simulink subsystem "PvtSubSys_LATC"  (R2020b)
settings: Solver=VariableStepAuto  StartTime=0.0  StopTime=10.0  RelTol=1e-3
undefined symbols (not defined in the file or in its folder): LCS_PLAN_PreViewIdxNum, LCS_PLAN_PreViewIdxSW_b, P_Global_CharSpd_ms, P_Global_SteeringAngleRatio, P_Global_WheelBase_m, P_LCS_DetNoOverRide_DrvTrq_TH, P_LCS_DetOverRide_DrvTrq_TH, P_LCS_ESS_AngleSlope_Limit, P_LCS_ESS_LogicTest_Enable, P_LCS_ESS_NotActiveFlgDelayTime, P_LCS_ESS_NotActiveFlgDelayTimeSW, P_LCS_ESS_SteerAngleErr, P_LCS_ESS_SteerAngleFilterTime, P_LCS_ESS_TarAngleFilterTime, P_LCS_ESSAngleSW, P_LCS_ESSOverrideTime1, P_LCS_ESSOverrideTime2, P_LCS_ESSOverrideTime3, P_LCS_ESSOverrideValue1, P_LCS_ESSOverrideValue2, P_LCS_IN_Offset_Test_SW, P_LCS_IN_Offset_Test_Value, P_LCS_LATC_AngleFilterTime_s, P_LCS_LATC_CurOffsetCurve_TabX_m, P_LCS_LATC_CurOffsetCurveFliterTime_Tab_s, P_LCS_LATC_CurOffsetVehicleSpdLimitValue_degs, P_LCS_LATC_DeltaEps_Tab_s, P_LCS_LATC_DxOffset_Sw, P_LCS_LATC_ELKAngleSlope_ratio, P_LCS_LATC_ELKMaxLatAcc_ms2, P_LCS_LATC_ESSA0Dis_TabX_m, P_LCS_LATC_ESSAddAngleSlope_Tab_degs, P_LCS_LATC_ESSAESAngleSlope_Tab_degs, P_LCS_LATC_ESSAngleSlope_ratio, P_LCS_LATC_ESSMaxLatAcc_ms2, P_LCS_LATC_LCAngleSlope_ratio, P_LCS_LATC_LCAngleSlope_Tab_degs, P_LCS_LATC_LCCancleMaxLatAcc_ms2, P_LCS_LATC_LCEcoAngleSlope_ratio, P_LCS_LATC_LCEcoAngleSlope_Tab_degs, P_LCS_LATC_LCEcoMaxLatAcc_ms2, P_LCS_LATC_LCKAngleSlope_ratio, P_LCS_LATC_LCKAngleSlope_Tab_degs, P_LCS_LATC_LCKIEAngleSlope_ratio, P_LCS_LATC_LCKIEAngleSlope_Tab_degs, P_LCS_LATC_LCKIEMaxLatAcc_ms2, P_LCS_LATC_LCKMaxLatAcc_ms2, P_LCS_LATC_LCNormalAngleSlope_ratio, P_LCS_LATC_LCNormalAngleSlope_Tab_degs, P_LCS_LATC_LCNormalMaxLatAcc_ms2, P_LCS_LATC_LCSportAngleSlope_ratio, P_LCS_LATC_LCSportAngleSlope_Tab_degs, P_LCS_LATC_LCSportMaxLatAcc_ms2, P_LCS_LATC_LKAAngleSlope_ratio, P_LCS_LATC_LKAAngleSlope_Tab_degs, P_LCS_LATC_LKAMaxLatAcc_ms2, P_LCS_LATC_MatrixQ1_st, P_LCS_LATC_MatrixQ3_st, P_LCS_LATC_MatrixR_st, P_LCS_LATC_MPCDeltaT_s ... (+70)
libraries: simulink x34
(part 2 of 5)

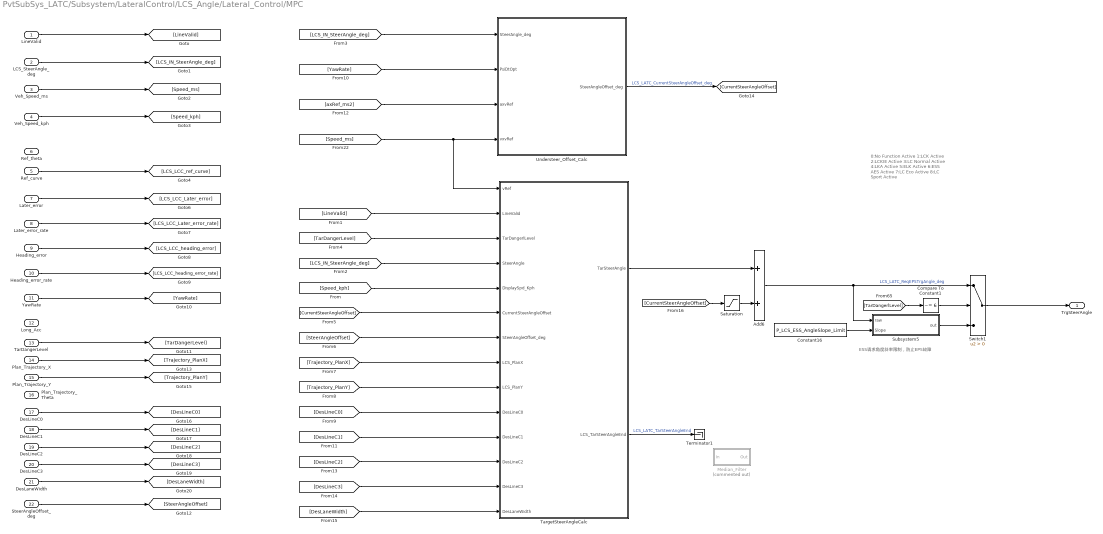
== system PvtSubSys_LATC/Subsystem/LateralControl/LCS_Angle/Lateral_Control/MPC ==
  note: ESS请求角度斜率限制，防止EPS故障
  note: 0:No Function Active
      | 1:LCK Active
      | 2:LCKIE Active
      | 3:LC Normal Active
      | 4:LKA Active
      | 5:ELK Active
      | 6:ESS AES Active
      | 7:LC Eco Active
      | 8:LC Sport Active
  LineValid : Inport
  LCS_SteerAngle_deg : Inport  Port=2
  Veh_Speed_ms : Inport  Port=3
  Veh_Speed_kph : Inport  Port=4
  Ref_curve : Inport  Port=5
  Ref_theta : Inport  Port=6
  Later_error : Inport  Port=7
  Later_error_rate : Inport  Port=8
  Heading_error : Inport  Port=9
  Heading_error_rate : Inport  Port=10
  YawRate : Inport  Port=11
  Long_Acc : Inport  Port=12
  TarDangerLevel : Inport  Port=13
  Plan_Trajectory_X : Inport  Port=14
  Plan_Trajectory_Y : Inport  Port=15
  Plan_Trajectory_Theta : Inport  Port=16
  DesLineC0 : Inport  Port=17
  DesLineC1 : Inport  Port=18
  DesLineC2 : Inport  Port=19
  DesLineC3 : Inport  Port=20
  DesLaneWidth : Inport  Port=21
  SteerAngleOffset_deg : Inport  Port=22
  Add6 : Sum  AccumDataTypeStr=single
  Compare To Constant1 : simulink/Logic and Bit Operations/Compare To Constant  relop=~=  const=6  OutDataTypeStr=boolean
  Constant16 : Constant  Value=P_LCS_ESS_AngleSlope_Limit  OutDataTypeStr=single
  Median_Filter : Subsystem  Commented=on
  Saturation : Saturate  UpperLimit=10  LowerLimit=-10
  Subsystem5 : Subsystem
  Switch1 : Switch  Criteria=u2 > Threshold
  TargetSteerAngleCalc : Subsystem
  Terminator1 : Terminator
  Understeer_Offset_Calc : Subsystem
  TrgSteerAngle : Outport  OutDataTypeStr=single
  wires:
  TarDangerLevel/1 -> [TarDangerLevel]
  YawRate/1 -> [YawRate]
  Later_error_rate/1 -> [LCS_LCC_Later_error_rate]
  Veh_Speed_kph/1 -> [Speed_kph]
  Veh_Speed_ms/1 -> [Speed_ms]
  [axRef_ms2] -> Understeer_Offset_Calc/3(axvRef)
  Understeer_Offset_Calc/1(SteerAngleOffset_deg) -> [CurrentSteerAngleOffset]  "LCS_LATC_CurrentSteerAngleOffset_deg"
  [YawRate] -> Understeer_Offset_Calc/2(PsiDtOpt)
  Heading_error_rate/1 -> [LCS_LCC_heading_error_rate]
  Heading_error/1 -> [LCS_LCC_heading_error]
  Ref_curve/1 -> [LCS_LCC_ref_curve]
  LCS_SteerAngle_deg/1 -> [LCS_IN_SteerAngle_deg]
  [LCS_IN_SteerAngle_deg] -> Understeer_Offset_Calc/1(SteerAngle_deg)
  Later_error/1 -> [LCS_LCC_Later_error]
  LineValid/1 -> [LineValid]
  [Speed_ms] -> TargetSteerAngleCalc/1(vRef), Understeer_Offset_Calc/4(vxvRef)
  [Speed_kph] -> TargetSteerAngleCalc/5(DisplaySpd_Kph)
  [LineValid] -> TargetSteerAngleCalc/2(LineValid)
  [LCS_IN_SteerAngle_deg] -> TargetSteerAngleCalc/4(SteerAngle)
  [TarDangerLevel] -> TargetSteerAngleCalc/3(TarDangerlLevel)
  [CurrentSteerAngleOffset] -> TargetSteerAngleCalc/6(CurrentSteerAngleOffset)
  [SteerAngleOffset] -> TargetSteerAngleCalc/7(SteerAngleOffset_deg)
  SteerAngleOffset_deg/1 -> [SteerAngleOffset]
  [Trajectory_PlanX] -> TargetSteerAngleCalc/8(LCS_PlanX)
  [Trajectory_PlanY] -> TargetSteerAngleCalc/9(LCS_PlanY)
  Plan_Trajectory_X/1 -> [Trajectory_PlanX]
  Plan_Trajectory_Y/1 -> [Trajectory_PlanY]
  [DesLineC0] -> TargetSteerAngleCalc/10(DesLineC0)
  [DesLineC1] -> TargetSteerAngleCalc/11(DesLineC1)
  [DesLineC2] -> TargetSteerAngleCalc/12(DesLineC2)
  [DesLineC3] -> TargetSteerAngleCalc/13(DesLineC3)
  [DesLaneWidth] -> TargetSteerAngleCalc/14(DesLaneWidth)
  DesLineC0/1 -> [DesLineC0]
  DesLineC1/1 -> [DesLineC1]
  DesLineC2/1 -> [DesLineC2]
  DesLineC3/1 -> [DesLineC3]
  DesLaneWidth/1 -> [DesLaneWidth]
  TargetSteerAngleCalc/2(LCS_TarSteerAngleEnd) -> Terminator1/1  "LCS_LATC_TarSteerAngleEnd"
  Subsystem5/1(out) -> Switch1/3
  Constant16/1 -> Subsystem5/2(Slope)
  [CurrentSteerAngleOffset] -> Saturation/1
  Saturation/1 -> Add6/2
  Add6/1 -> Subsystem5/1(raw), Switch1/1  "LCS_LATC_ReqEPSTrgAngle_deg"
  Compare To Constant1/1 -> Switch1/2
  [TarDangerlLevel] -> Compare To Constant1/1
  Switch1/1 -> TrgSteerAngle/1
  TargetSteerAngleCalc/1(TarSteerAngle) -> Add6/1

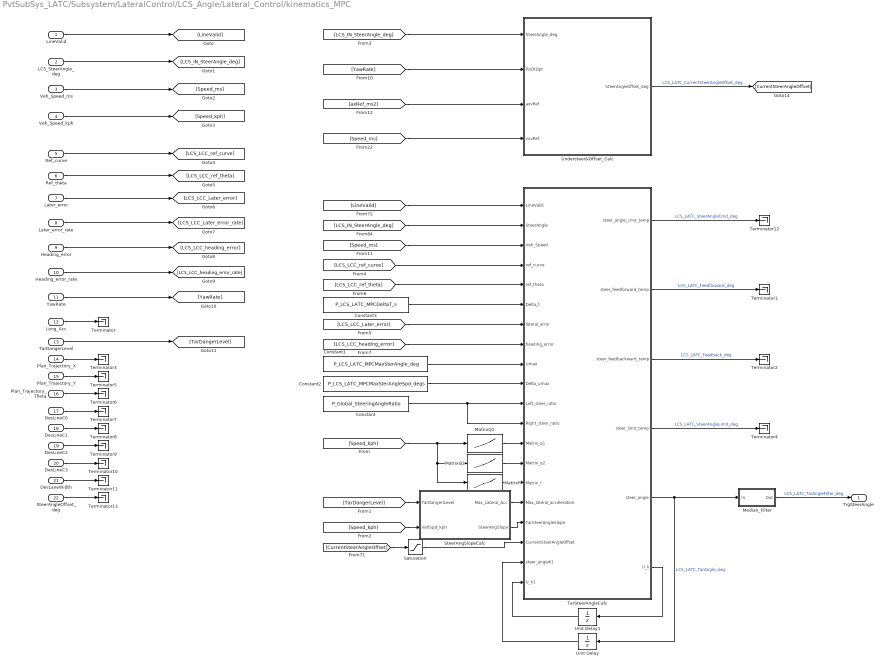
== system PvtSubSys_LATC/Subsystem/LateralControl/LCS_Angle/Lateral_Control/kinematics_MPC ==
  LineValid : Inport
  LCS_SteerAngle_deg : Inport  Port=2
  Veh_Speed_ms : Inport  Port=3
  Veh_Speed_kph : Inport  Port=4
  Ref_curve : Inport  Port=5
  Ref_theta : Inport  Port=6
  Later_error : Inport  Port=7
  Later_error_rate : Inport  Port=8
  Heading_error : Inport  Port=9
  Heading_error_rate : Inport  Port=10
  YawRate : Inport  Port=11
  Long_Acc : Inport  Port=12
  TarDangerLevel : Inport  Port=13
  Plan_Trajectory_X : Inport  Port=14
  Plan_Trajectory_Y : Inport  Port=15
  Plan_Trajectory_Theta : Inport  Port=16
  DesLineC0 : Inport  Port=17
  DesLineC1 : Inport  Port=18
  DesLineC2 : Inport  Port=19
  DesLineC3 : Inport  Port=20
  DesLaneWidth : Inport  Port=21
  SteerAngleOffset_deg : Inport  Port=22
  Constant : Constant  Value=P_Global_SteeringAngleRatio  OutDataTypeStr=single
  Constant1 : Constant  Value=P_LCS_LATC_MPCMaxSterAngle_deg  OutDataTypeStr=single
  Constant2 : Constant  Value=P_LCS_LATC_MPCMaxSterAngleSpd_degs  OutDataTypeStr=single
  Constant3 : Constant  Value=P_LCS_LATC_MPCDeltaT_s  OutDataTypeStr=single
  MatrixQ1 : Lookup_n-D  NumberOfTableDimensions=1  BreakpointsForDimension1=P_LCS_VehicleSpd_TabX_Kph  Table=P_LCS_LATC_MPCMatrixQ1_st  ExtrapMethod=Clip  UseLastTableValue=on  InternalRulePriority=Speed  RndMeth=Simplest  InputSameDT=on
  MatrixQ2 : Lookup_n-D  NumberOfTableDimensions=1  BreakpointsForDimension1=P_LCS_VehicleSpd_TabX_Kph  Table=P_LCS_LATC_MPCMatrixQ2_st  ExtrapMethod=Clip  UseLastTableValue=on  InternalRulePriority=Speed  RndMeth=Simplest  InputSameDT=on
  MatrixR : Lookup_n-D  NumberOfTableDimensions=1  BreakpointsForDimension1=P_LCS_VehicleSpd_TabX_Kph  Table=P_LCS_LATC_MPCMatrixR_st  ExtrapMethod=Clip  UseLastTableValue=on  InternalRulePriority=Speed  RndMeth=Simplest  InputSameDT=on
  Median_Filter : Subsystem
  Saturation : Saturate  UpperLimit=8  LowerLimit=-8  OutDataTypeStr=single
  SteerAngSlopeCalc : Subsystem
  TarSteerAngleCalc : MATLAB Function  TreatAsAtomicUnit=on
  Terminator{,1..13} (14 alike) : Terminator
  Understeer&Offset_Calc : Subsystem
  Unit Delay : UnitDelay  SampleTime=-1  HasFrameUpgradeWarning=on
  Unit Delay1 : UnitDelay  SampleTime=-1  HasFrameUpgradeWarning=on
  TrgSteerAngle : Outport  OutDataTypeStr=single
  wires:
  [LCS_LCC_ref_theta] -> TarSteerAngleCalc/5(ref_theta)
  Ref_theta/1 -> [LCS_LCC_ref_theta]
  Constant3/1 -> TarSteerAngleCalc/6(Delta_t)
  Constant2/1 -> TarSteerAngleCalc/10(Delta_umax)
  Constant1/1 -> TarSteerAngleCalc/9(Umax)
  [LCS_LCC_ref_curve] -> TarSteerAngleCalc/4(ref_curve)
  Unit Delay1/1 -> TarSteerAngleCalc/20(U_k1)
  TarSteerAngleCalc/6(U_k) -> Unit Delay1/1
  Heading_error_rate/1 -> [LCS_LCC_heading_error_rate]
  Long_Acc/1 -> Terminator/1
  Constant/1 -> TarSteerAngleCalc/12(Right_steer_ratio), TarSteerAngleCalc/11(Left_steer_ratio)
  [Speed_kph] -> MatrixQ2/1, MatrixR/1, MatrixQ1/1
  TarSteerAngleCalc/4(steer_limit_temp) -> Terminator4/1  "LCS_LATC_SteerAngleLimit_deg"
  DesLineC3/1 -> Terminator10/1
  MatrixR/1 -> TarSteerAngleCalc/15(Matrix_r)
  [LCS_LCC_Later_error] -> TarSteerAngleCalc/7(lateral_error)
  TarSteerAngleCalc/3(steer_feedbackward_temp) -> Terminator2/1  "LCS_LATC_Feedback_deg"
  [LineValid] -> TarSteerAngleCalc/1(LineValid)
  [Speed_kph] -> SteerAngSlopeCalc/2(VehSpd_kph)
  LCS_SteerAngle_deg/1 -> [LCS_IN_SteerAngle_deg]
  TarSteerAngleCalc/5(steer_angle) -> Median_Filter/1(In), Unit Delay/1  "LCS_LATC_TarAngle_deg"
  [Speed_ms] -> Understeer&Offset_Calc/4(vxvRef)
  Saturation/1 -> TarSteerAngleCalc/18(CurrentSteerAngleOffset)
  [CurrentSteerAngleOffset] -> Saturation/1
  TarDangerLevel/1 -> [TarDangerLevel]
  [LCS_LCC_heading_error] -> TarSteerAngleCalc/8(heading_error)
  [LCS_IN_SteerAngle_deg] -> TarSteerAngleCalc/2(SteerAngle)
  TarSteerAngleCalc/2(steer_feedforward_temp) -> Terminator1/1  "LCS_LATC_Feedforward_deg"
  Median_Filter/1(Out) -> TrgSteerAngle/1  "LCS_LATC_TarAngleFilter_deg"
  [Speed_ms] -> TarSteerAngleCalc/3(Veh_Speed)
  Veh_Speed_ms/1 -> [Speed_ms]
  MatrixQ2/1 -> TarSteerAngleCalc/14(Matrix_q2)
  Later_error/1 -> [LCS_LCC_Later_error]
  Heading_error/1 -> [LCS_LCC_heading_error]
  [YawRate] -> Understeer&Offset_Calc/2(PsiDtOpt)
  LineValid/1 -> [LineValid]
  SteerAngSlopeCalc/2(SteerAngSlope) -> TarSteerAngleCalc/17(TarSteerAngleSlope)
  [LCS_IN_SteerAngle_deg] -> Understeer&Offset_Calc/1(SteerAngle_deg)
  [TarDangerLevel] -> SteerAngSlopeCalc/1(TarDangerlLevel)
  TarSteerAngleCalc/1(steer_angle_cmd_temp) -> Terminator12/1  "LCS_LATC_SteerAngleCmd_deg"
  DesLineC0/1 -> Terminator7/1
  MatrixQ1/1 -> TarSteerAngleCalc/13(Matrix_q1)
  YawRate/1 -> [YawRate]
  [axRef_ms2] -> Understeer&Offset_Calc/3(axvRef)
  Veh_Speed_kph/1 -> [Speed_kph]
  SteerAngSlopeCalc/1(Max_Lateral_Acc) -> TarSteerAngleCalc/16(Max_lateral_acceleration)
  Plan_Trajectory_Theta/1 -> Terminator6/1
  DesLineC2/1 -> Terminator9/1
  DesLineC1/1 -> Terminator8/1
  Later_error_rate/1 -> [LCS_LCC_Later_error_rate]
  Plan_Trajectory_Y/1 -> Terminator5/1
  DesLaneWidth/1 -> Terminator11/1
  Ref_curve/1 -> [LCS_LCC_ref_curve]
  SteerAngleOffset_deg/1 -> Terminator13/1
  Plan_Trajectory_X/1 -> Terminator3/1
  Understeer&Offset_Calc/1(SteerAngleOffset_deg) -> [CurrentSteerAngleOffset]  "LCS_LATC_CurrentSteerAngleOffset_deg"
  Unit Delay/1 -> TarSteerAngleCalc/19(steer_angleK1)

== system PvtSubSys_LATC/Subsystem/LateralControl/LCS_Angle/Motion_Planning/CartesianTrajectory ==
  DesLineValid : Inport
  DesLineC0 : Inport  Port=2
  DesLineC1 : Inport  Port=3
  DesLineC2 : Inport  Port=4
  DesLineC3 : Inport  Port=5
  Veh_Speed_ms : Inport  Port=6
  YawRate : Inport  Port=7
  Veh_Speed_kph : Inport  Port=8
  TarDangerLevel : Inport  Port=9
  Long_Acc : Inport  Port=10
  kapEgo : Inport  Port=11
  Constant : Constant  Value=LCS_PLAN_PreViewIdxSW_b
  Constant1 : Constant  Value=LCS_PLAN_PreViewIdxNum
  DesLineC4 : InportShadow  Port=5
  DesLineC5 : InportShadow  Port=4
  DesLineC6 : InportShadow  Port=2
  FrenetTrajectory : MATLAB Function  TreatAsAtomicUnit=on
  Subsystem1 : Subsystem
  Terminator : Terminator
  Veh_Speed_ms1 : InportShadow  Port=6
  PlanX : Outport
  PlanY : Outport  Port=2
  PlanTheta : Outport  Port=3
  idx : Outport  Port=4
  PreviewX : Outport  Port=5
  PreviewY : Outport  Port=6
  PreviewTheta : Outport  Port=7
  numTraj : Outport  Port=8
  ref_curvature : Outport  Port=9
  ref_theta : Outport  Port=10
  lateral_error : Outport  Port=11
  lateral_error_rate : Outport  Port=12
  heading_error : Outport  Port=13
  heading_error_rate : Outport  Port=14
  wires:
  Constant1/1 -> FrenetTrajectory/13(PreViewIdxNum)
  Constant/1 -> FrenetTrajectory/12(PreViewIdxSW)
  FrenetTrajectory/10(ref_theta) -> ref_theta/1
  DesLineValid/1 -> Terminator/1
  Subsystem1/3(Min_Plan_Dis) -> FrenetTrajectory/9(Min_Plan_Dis)
  kapEgo/1 -> FrenetTrajectory/11(kapEgo)
  DesLineC0/1 -> FrenetTrajectory/1(A0)
  DesLineC1/1 -> FrenetTrajectory/2(A1)
  DesLineC2/1 -> FrenetTrajectory/3(A2)
  DesLineC3/1 -> FrenetTrajectory/4(A3)
  Veh_Speed_ms/1 -> FrenetTrajectory/5(Veh_Speed)
  YawRate/1 -> FrenetTrajectory/6(YawRate)
  FrenetTrajectory/1(PlanX) -> PlanX/1
  FrenetTrajectory/2(PlanY) -> PlanY/1
  FrenetTrajectory/3(PlanTheta) -> PlanTheta/1
  FrenetTrajectory/4(idx) -> idx/1
  FrenetTrajectory/5(PreviewX) -> PreviewX/1
  FrenetTrajectory/6(PreviewY) -> PreviewY/1
  FrenetTrajectory/7(PreviewTheta) -> PreviewTheta/1
  FrenetTrajectory/8(numTraj) -> numTraj/1
  FrenetTrajectory/9(ref_curvature) -> ref_curvature/1
  FrenetTrajectory/11(lateral_error) -> lateral_error/1
  FrenetTrajectory/12(lateral_error_rate) -> lateral_error_rate/1
  FrenetTrajectory/13(heading_error) -> heading_error/1
  FrenetTrajectory/14(heading_error_rate) -> heading_error_rate/1
  Long_Acc/1 -> FrenetTrajectory/10(axEgo)
  Subsystem1/1(Preview_T) -> FrenetTrajectory/7(PreView_T)
  Subsystem1/2(AyDtLimit) -> FrenetTrajectory/8(AyDtLimit)
  TarDangerLevel/1 -> Subsystem1/1(TarDangerLevel)
  Veh_Speed_ms1/1 -> Subsystem1/3(VehSpd_ms)
  Veh_Speed_kph/1 -> Subsystem1/2(Spd_kph)
  DesLineC6/1 -> Subsystem1/4(LCS_IN_desLaneA0)
  DesLineC5/1 -> Subsystem1/5(LCS_IN_desLaneA2)
  DesLineC4/1 -> Subsystem1/6(LCS_IN_desLaneA3)

== system PvtSubSys_LATC/Subsystem/LateralControl/LCS_Angle/Motion_Planning/CartesianTrajectory_MPC ==
  DesLineValid : Inport
  DesLineC0 : Inport  Port=2
  DesLineC1 : Inport  Port=3
  DesLineC2 : Inport  Port=4
  DesLineC3 : Inport  Port=5
  Veh_Speed_ms : Inport  Port=6
  YawRate : Inport  Port=7
  Veh_Speed_kph : Inport  Port=8
  TarDangerLevel : Inport  Port=9
  Long_Acc : Inport  Port=10
  kapEgo : Inport  Port=11
  CartesianTrajectory : MATLAB Function  TreatAsAtomicUnit=on
  Constant10 : Constant  Value=P_LCS_PLAN_DisFac_Tab_ratio  OutDataTypeStr=single
  Constant2 : Constant  Value=P_LCS_PLAN_MinDis_m  OutDataTypeStr=single
  Ground{,1..10} (11 alike) : Ground
  Subsystem : Subsystem
  Terminator{2..7,9..10} (8 alike) : Terminator
  Veh_Speed_ms1 : InportShadow  Port=6
  PlanX : Outport
  PlanY : Outport  Port=2
  PlanTheta : Outport  Port=3
  idx : Outport  Port=4
  PreviewX : Outport  Port=5
  PreviewY : Outport  Port=6
  PreviewTheta : Outport  Port=7
  numTraj : Outport  Port=8
  ref_curvature : Outport  Port=9
  ref_theta : Outport  Port=10
  lateral_error : Outport  Port=11
  lateral_error_rate : Outport  Port=12
  heading_error : Outport  Port=13
  heading_error_rate : Outport  Port=14
  wires:
  Ground10/1 -> ref_theta/1
  CartesianTrajectory/6(planLength) -> Terminator10/1  "LCS_LATC_PlanLength"
  CartesianTrajectory/5(LoopNum) -> numTraj/1
  CartesianTrajectory/7(Ay) -> Terminator4/1
  CartesianTrajectory/11(break_AyDtValue) -> Terminator6/1
  CartesianTrajectory/2(planY) -> PlanY/1
  CartesianTrajectory/1(planX) -> PlanX/1
  CartesianTrajectory/3(planValid) -> Terminator9/1
  CartesianTrajectory/8(AyDt) -> Terminator5/1  "LCS_LATC_PlanAyDt"
  CartesianTrajectory/9(break_Flg) -> Terminator3/1
  CartesianTrajectory/4(planT) -> Terminator7/1  "LCS_LATC_PlanT"
  CartesianTrajectory/10(break_AyValue) -> Terminator2/1
  Ground/1 -> PlanTheta/1
  Ground1/1 -> idx/1
  Ground2/1 -> PreviewX/1
  Ground3/1 -> PreviewY/1
  Ground4/1 -> PreviewTheta/1
  Ground5/1 -> ref_curvature/1
  Ground6/1 -> lateral_error/1
  Ground7/1 -> lateral_error_rate/1
  Ground8/1 -> heading_error/1
  Ground9/1 -> heading_error_rate/1
  Veh_Speed_ms/1 -> CartesianTrajectory/1(vEgo)
  DesLineC0/1 -> Subsystem/4(DesLineC0), CartesianTrajectory/8(TarLineC0)
  DesLineC1/1 -> Subsystem/5(DesLineC1), CartesianTrajectory/7(TarLineC1)
  DesLineC2/1 -> Subsystem/6(DesLineC2), CartesianTrajectory/6(TarLineC2)
  DesLineC3/1 -> Subsystem/7(DesLineC3), CartesianTrajectory/5(TarLineC3)
  kapEgo/1 -> CartesianTrajectory/2(kapEgo)
  Long_Acc/1 -> CartesianTrajectory/3(axEgo)
  DesLineValid/1 -> CartesianTrajectory/4(TarLineValid)
  Subsystem/1(Plan_ayDtLimit) -> CartesianTrajectory/9(ayDtLimit)
  Subsystem/2(Plan_FinalpreDis) -> CartesianTrajectory/10(PreDis)
  Constant10/1 -> CartesianTrajectory/11(Dis_Fac)
  Constant2/1 -> CartesianTrajectory/12(Min_PlanDis)
  TarDangerLevel/1 -> Subsystem/1(TarDangerlLevel)
  Veh_Speed_ms1/1 -> Subsystem/3(Veh_Speed_ms)
  Veh_Speed_kph/1 -> Subsystem/2(vDisplay_Kph)

== system PvtSubSys_LATC/Subsystem/LateralControl/LCS_Angle/Motion_Planning/FrenetTrajectory ==
  DesLineValid : Inport
  DesLineC0 : Inport  Port=2
  DesLineC1 : Inport  Port=3
  DesLineC2 : Inport  Port=4
  DesLineC3 : Inport  Port=5
  Veh_Speed_ms : Inport  Port=6
  YawRate : Inport  Port=7
  Veh_Speed_kph : Inport  Port=8
  TarDangerLevel : Inport  Port=9
  Long_Acc : Inport  Port=10
  kapEgo : Inport  Port=11
  Constant : Constant  Value=LCS_PLAN_PreViewIdxSW_b
  Constant1 : Constant  Value=LCS_PLAN_PreViewIdxNum
  DesLineC4 : InportShadow  Port=2
  DesLineC5 : InportShadow  Port=4
  DesLineC6 : InportShadow  Port=5
  FrenetTrajectory : MATLAB Function  TreatAsAtomicUnit=on
  Subsystem : Subsystem
  Terminator : Terminator
  Terminator1 : Terminator
  Terminator2 : Terminator
  Veh_Speed_ms1 : InportShadow  Port=6
  PlanX : Outport
  PlanY : Outport  Port=2
  PlanTheta : Outport  Port=3
  idx : Outport  Port=4
  PreviewX : Outport  Port=5
  PreviewY : Outport  Port=6
  PreviewTheta : Outport  Port=7
  numTraj : Outport  Port=8
  ref_curvature : Outport  Port=9
  ref_theta : Outport  Port=10
  lateral_error : Outport  Port=11
  lateral_error_rate : Outport  Port=12
  heading_error : Outport  Port=13
  heading_error_rate : Outport  Port=14
  wires:
  Constant1/1 -> FrenetTrajectory/11(PreViewIdxNum)
  Constant/1 -> FrenetTrajectory/10(PreViewIdxSW)
  FrenetTrajectory/10(ref_theta) -> ref_theta/1
  DesLineValid/1 -> Terminator2/1
  Subsystem/3(Min_Plan_Dis) -> FrenetTrajectory/9(Min_Plan_Dis)
  kapEgo/1 -> Terminator1/1
  DesLineC6/1 -> Subsystem/6(LCS_IN_desLaneA3)
  DesLineC5/1 -> Subsystem/5(LCS_IN_desLaneA2)
  DesLineC4/1 -> Subsystem/4(LCS_IN_desLaneA0)
  Veh_Speed_kph/1 -> Subsystem/2(Spd_kph)
  Veh_Speed_ms1/1 -> Subsystem/3(VehSpd_ms)
  TarDangerLevel/1 -> Subsystem/1(TarDangerLevel)
  Subsystem/2(AyDtLimit) -> FrenetTrajectory/8(AyDtLimit)
  Subsystem/1(Preview_T) -> FrenetTrajectory/7(PreView_T)
  Long_Acc/1 -> Terminator/1
  FrenetTrajectory/14(heading_error_rate) -> heading_error_rate/1
  FrenetTrajectory/13(heading_error) -> heading_error/1
  FrenetTrajectory/12(lateral_error_rate) -> lateral_error_rate/1
  FrenetTrajectory/11(lateral_error) -> lateral_error/1
  FrenetTrajectory/9(ref_curvature) -> ref_curvature/1
  FrenetTrajectory/8(numTraj) -> numTraj/1
  FrenetTrajectory/7(PreviewTheta) -> PreviewTheta/1
  FrenetTrajectory/6(PreviewY) -> PreviewY/1
  FrenetTrajectory/5(PreviewX) -> PreviewX/1
  FrenetTrajectory/4(idx) -> idx/1
  FrenetTrajectory/3(PlanTheta) -> PlanTheta/1
  FrenetTrajectory/2(PlanY) -> PlanY/1
  FrenetTrajectory/1(PlanX) -> PlanX/1
  YawRate/1 -> FrenetTrajectory/6(YawRate)
  Veh_Speed_ms/1 -> FrenetTrajectory/5(Veh_Speed)
  DesLineC3/1 -> FrenetTrajectory/4(A3)
  DesLineC2/1 -> FrenetTrajectory/3(A2)
  DesLineC1/1 -> FrenetTrajectory/2(A1)
  DesLineC0/1 -> FrenetTrajectory/1(A0)

== system PvtSubSys_LATC/Subsystem/LateralControl/LCS_Angle/Motion_Planning/FrenetTrajectory_Lateral ==
  DesLineValid : Inport
  DesLineC0 : Inport  Port=2
  DesLineC1 : Inport  Port=3
  DesLineC2 : Inport  Port=4
  DesLineC3 : Inport  Port=5
  Veh_Speed_ms : Inport  Port=6
  YawRate : Inport  Port=7
  Veh_Speed_kph : Inport  Port=8
  TarDangerLevel : Inport  Port=9
  Long_Acc : Inport  Port=10
  kapEgo : Inport  Port=11
  Constant : Constant  Value=LCS_PLAN_PreViewIdxSW_b
  Constant1 : Constant  Value=LCS_PLAN_PreViewIdxNum
  DesLineC4 : InportShadow  Port=2
  DesLineC5 : InportShadow  Port=4
  DesLineC6 : InportShadow  Port=5
  FrenetTrajectory_Lateral : MATLAB Function  TreatAsAtomicUnit=on
  Subsystem1 : Subsystem
  Terminator : Terminator
  Terminator1 : Terminator
  Terminator2 : Terminator
  Veh_Speed_ms1 : InportShadow  Port=6
  PlanX : Outport
  PlanY : Outport  Port=2
  PlanTheta : Outport  Port=3
  idx : Outport  Port=4
  PreviewX : Outport  Port=5
  PreviewY : Outport  Port=6
  PreviewTheta : Outport  Port=7
  numTraj : Outport  Port=8
  ref_curvature : Outport  Port=9
  ref_theta : Outport  Port=10
  lateral_error : Outport  Port=11
  lateral_error_rate : Outport  Port=12
  heading_error : Outport  Port=13
  heading_error_rate : Outport  Port=14
  wires:
  Constant1/1 -> FrenetTrajectory_Lateral/12(PreViewIdxNum)
  Constant/1 -> FrenetTrajectory_Lateral/11(PreViewIdxSW)
  FrenetTrajectory_Lateral/10(ref_theta) -> ref_theta/1
  Subsystem1/3(Min_Plan_Dis) -> FrenetTrajectory_Lateral/10(Min_Plan_Dis)
  DesLineValid/1 -> Terminator2/1
  kapEgo/1 -> Terminator1/1
  DesLineC6/1 -> Subsystem1/6(LCS_IN_desLaneA3)
  DesLineC5/1 -> Subsystem1/5(LCS_IN_desLaneA2)
  DesLineC0/1 -> FrenetTrajectory_Lateral/1(A0)
  DesLineC1/1 -> FrenetTrajectory_Lateral/2(A1)
  DesLineC2/1 -> FrenetTrajectory_Lateral/3(A2)
  DesLineC3/1 -> FrenetTrajectory_Lateral/4(A3)
  Veh_Speed_ms/1 -> FrenetTrajectory_Lateral/5(Veh_Speed)
  YawRate/1 -> FrenetTrajectory_Lateral/6(YawRate)
  FrenetTrajectory_Lateral/1(PlanX) -> PlanX/1
  FrenetTrajectory_Lateral/2(PlanY) -> PlanY/1
  FrenetTrajectory_Lateral/3(PlanTheta) -> PlanTheta/1
  FrenetTrajectory_Lateral/4(idx) -> idx/1
  FrenetTrajectory_Lateral/5(PreviewX) -> PreviewX/1
  FrenetTrajectory_Lateral/6(PreviewY) -> PreviewY/1
  FrenetTrajectory_Lateral/7(PreviewTheta) -> PreviewTheta/1
  FrenetTrajectory_Lateral/8(numTraj) -> numTraj/1
  FrenetTrajectory_Lateral/9(ref_curvature) -> ref_curvature/1
  FrenetTrajectory_Lateral/11(lateral_error) -> lateral_error/1
  FrenetTrajectory_Lateral/12(lateral_error_rate) -> lateral_error_rate/1
  FrenetTrajectory_Lateral/13(heading_error) -> heading_error/1
  FrenetTrajectory_Lateral/14(heading_error_rate) -> heading_error_rate/1
  Long_Acc/1 -> Terminator/1
  Subsystem1/1(Preview_T) -> FrenetTrajectory_Lateral/8(PreView_T)
  Subsystem1/2(AyDtLimit) -> FrenetTrajectory_Lateral/9(AyDtLimit)
  TarDangerLevel/1 -> FrenetTrajectory_Lateral/7(TarDangerlLevel), Subsystem1/1(TarDangerLevel)
  Veh_Speed_ms1/1 -> Subsystem1/3(VehSpd_ms)
  Veh_Speed_kph/1 -> Subsystem1/2(Spd_kph)
  DesLineC4/1 -> Subsystem1/4(LCS_IN_desLaneA0)

== system PvtSubSys_LATC/Subsystem/LateralControl/LCS_Angle/OverRideDetect/LP filter4 ==
  note: deltaT = time(signal) - time(signal[-1]);
      |    alpha = 1/(1/2/pi/deltaT/fc + 1);
      |    result = alpha * signal + (1 - alpha) * LastValue;
  Raw : Inport
  TorqFilterTime : Inport  Port=2
  enable : Inport  Port=3
  Add : Sum
  Add1 : Sum  Inputs=+-
  Data Type Conversion : DataTypeConversion  OutDataTypeStr=single
  Memory2 : Memory  InheritSampleTime=on
  Product2 : Product  Inputs=*/  RndMeth=Zero
  Product3 : Product  RndMeth=Zero
  Product4 : Product  Inputs=*//  RndMeth=Zero
  Product5 : Product  RndMeth=Zero
  Sum1 : Sum  Inputs=++|
  Switch1 : Switch  Criteria=u2 ~= 0
  Weight/N1 : Constant  Value=0.1591549431  OutDataTypeStr=single
  Weight/N2 : Constant  OutDataTypeStr=single
  Weight/N3 : Constant  Value=0.02  OutDataTypeStr=single
  output : Outport
  wires:
  TorqFilterTime/1 -> Product4/3
  Product4/1 -> Add/1
  Weight/N3/1 -> Product4/2
  Memory2/1 -> Data Type Conversion/1
  enable/1 -> Switch1/2
  Raw/1 -> Product3/2, Switch1/3
  Switch1/1 -> output/1, Memory2/1
  Weight/N1/1 -> Product4/1
  Weight/N2/1 -> Add1/1, Product2/1, Add/2
  Add/1 -> Product2/2
  Product2/1 -> Product3/1, Add1/2
  Product3/1 -> Sum1/2
  Add1/1 -> Product5/2
  Product5/1 -> Sum1/1
  Sum1/1 -> Switch1/1
  Data Type Conversion/1 -> Product5/1

== system PvtSubSys_LATC/Subsystem/LateralControl/LCS_Angle/OverRideDetect/Subsystem17 ==
  In1 : Inport
  Add : Sum
  Constant : Constant  Value=Ts
  Constant1 : Constant  Value=0
  Constant2 : Constant  Value=Max
  Max : MinMax  Inputs=2
  Switch : Switch  Criteria=u2 ~= 0
  Unit Delay : UnitDelay  SampleTime=-1  HasFrameUpgradeWarning=on
  Out1 : Outport
  wires:
  Switch/1 -> Max/1
  Constant2/1 -> Max/2
  Max/1 -> Out1/1, Unit Delay/1
  Add/1 -> Switch/1
  Constant1/1 -> Switch/3
  Constant/1 -> Add/2
  In1/1 -> Switch/2
  Unit Delay/1 -> Add/1

== system PvtSubSys_LATC/Subsystem/LateralControl/LCS_Angle/OverRideDetect/Subsystem4 ==
  In1 : Inport
  Add : Sum
  Constant : Constant  Value=Ts
  Constant1 : Constant  Value=0
  Constant2 : Constant  Value=Max
  Max : MinMax  Inputs=2
  Switch : Switch  Criteria=u2 ~= 0
  Unit Delay : UnitDelay  SampleTime=-1  HasFrameUpgradeWarning=on
  Out1 : Outport
  wires:
  Unit Delay/1 -> Add/1
  In1/1 -> Switch/2
  Constant/1 -> Add/2
  Constant1/1 -> Switch/3
  Add/1 -> Switch/1
  Max/1 -> Unit Delay/1, Out1/1
  Constant2/1 -> Max/2
  Switch/1 -> Max/1

== system PvtSubSys_LATC/Subsystem/LateralControl/LCS_Angle/Lateral_Control/Dynamic_Model_LQR/Median_Filter ==
  In : Inport
  Constant11 : Constant  Value=P_LCS_LATC_TarAngleFliterWindowSize - single(2)  OutDataTypeStr=single
  Divide1 : Product  Inputs=*/
  Max of Elements1 : MinMax  Function=max
  MinMax2 : MinMax
  Minus1 : Sum  Inputs=--+
  Sum of Elements1 : Sum  Inputs=+
  Tapped Delay1 : simulink/Discrete/Tapped Delay  vinit=0.0  samptime=-1  NumDelays=P_LCS_LATC_TarAngleFliterWindowSize-1  DelayOrder=Newest  includeCurrent=on
  Out : Outport
  wires:
  Max of Elements1/1 -> Minus1/2
  Divide1/1 -> Out/1
  Minus1/1 -> Divide1/1
  In/1 -> Tapped Delay1/1
  MinMax2/1 -> Minus1/1
  Sum of Elements1/1 -> Minus1/3
  Tapped Delay1/1 -> Max of Elements1/1, MinMax2/1, Sum of Elements1/1
  Constant11/1 -> Divide1/2

== system PvtSubSys_LATC/Subsystem/LateralControl/LCS_Angle/Lateral_Control/Dynamic_Model_LQR/SteerAngSlopeCalc ==
  note: 换道状态切换检测
  note: 0:No Function Active
      | 1:LCK Active
      | 2:LCKIE Active
      | 3:LC Normal Active
      | 4:LKA Active
      | 5:ELK Active
      | 6:ESS AES Active
      | 7:LC Eco Active
      | 8:LC Sport Active
      | 9:LC cancel
  TarDangerlLevel : Inport
  VehSpd_kph : Inport  Port=2
  Constant : Constant  Value=0.4  OutDataTypeStr=single
  Constant1 : Constant  Value=1.5  OutDataTypeStr=single
  Constant2 : Constant  Value=P_LCS_LATC_StateHoldTime_st  OutDataTypeStr=uint16
  Constant3 : Constant  Value=0.02
  Constant4 : Constant  Value=0.4  OutDataTypeStr=single
  Constant5 : Constant  Value=1.5  OutDataTypeStr=single
  Data Type Conversion : DataTypeConversion  OutDataTypeStr=single
  Data Type Conversion1 : DataTypeConversion  OutDataTypeStr=single
  ELK Active : Lookup_n-D  NumberOfTableDimensions=1  BreakpointsForDimension1=P_LCS_VehicleSpd_TabX_Kph  Table=P_LCS_LATC_ELKAngleSlope_ratio  ExtrapMethod=Clip  InternalRulePriority=Speed  RndMeth=Simplest  InputSameDT=on
  ELK_MaxAy : Lookup_n-D  NumberOfTableDimensions=1  BreakpointsForDimension1=P_LCS_VehicleSpd_TabX_Kph  Table=P_LCS_LATC_ELKMaxLatAcc_ms2  ExtrapMethod=Clip  InternalRulePriority=Speed  RndMeth=Simplest  InputSameDT=on
  ESS AES Active : Lookup_n-D  NumberOfTableDimensions=1  BreakpointsForDimension1=P_LCS_VehicleSpd_TabX_Kph  Table=P_LCS_LATC_ESSAngleSlope_ratio  ExtrapMethod=Clip  InternalRulePriority=Speed  RndMeth=Simplest  InputSameDT=on
  ESS AES_MaxAy : Lookup_n-D  NumberOfTableDimensions=1  BreakpointsForDimension1=P_LCS_VehicleSpd_TabX_Kph  Table=P_LCS_LATC_ESSMaxLatAcc_ms2  ExtrapMethod=Clip  InternalRulePriority=Speed  RndMeth=Simplest  InputSameDT=on
  LC Cancel : Lookup_n-D  NumberOfTableDimensions=1  BreakpointsForDimension1=P_LCS_VehicleSpd_TabX_Kph  Table=P_LCS_LATC_LCAngleSlope_ratio  ExtrapMethod=Clip  InternalRulePriority=Speed  RndMeth=Simplest  InputSameDT=on
  LCK/IE TO LC_Eco : Lookup_n-D  NumberOfTableDimensions=1  BreakpointsForDimension1=P_LCS_VehicleSpd_TabX_Kph  Table=P_LCS_LATC_LCEcoAngleSlope_ratio  ExtrapMethod=Clip  InternalRulePriority=Speed  RndMeth=Simplest  InputSameDT=on
  LCK/IE TO LC_Nomal : Lookup_n-D  NumberOfTableDimensions=1  BreakpointsForDimension1=P_LCS_VehicleSpd_TabX_Kph  Table=P_LCS_LATC_LCNormalAngleSlope_ratio  ExtrapMethod=Clip  InternalRulePriority=Speed  RndMeth=Simplest  InputSameDT=on
  LCK/IE TO LC_Sport : Lookup_n-D  NumberOfTableDimensions=1  BreakpointsForDimension1=P_LCS_VehicleSpd_TabX_Kph  Table=P_LCS_LATC_LCSportAngleSlope_ratio  ExtrapMethod=Clip  InternalRulePriority=Speed  RndMeth=Simplest  InputSameDT=on
  LCKIEMaxAy : Lookup_n-D  NumberOfTableDimensions=1  BreakpointsForDimension1=P_LCS_VehicleSpd_TabX_Kph  Table=P_LCS_LATC_LCKIEMaxLatAcc_ms2  ExtrapMethod=Clip  InternalRulePriority=Speed  RndMeth=Simplest  InputSameDT=on
  LCKIE_Active : Lookup_n-D  NumberOfTableDimensions=1  BreakpointsForDimension1=P_LCS_VehicleSpd_TabX_Kph  Table=P_LCS_LATC_LCKIEAngleSlope_ratio  ExtrapMethod=Clip  InternalRulePriority=Speed  RndMeth=Simplest  InputSameDT=on
  LCKMaxAy : Lookup_n-D  NumberOfTableDimensions=1  BreakpointsForDimension1=P_LCS_VehicleSpd_TabX_Kph  Table=P_LCS_LATC_LCKMaxLatAcc_ms2  ExtrapMethod=Clip  InternalRulePriority=Speed  RndMeth=Simplest  InputSameDT=on
  LCNomal_MaxAy : Lookup_n-D  NumberOfTableDimensions=1  BreakpointsForDimension1=P_LCS_VehicleSpd_TabX_Kph  Table=P_LCS_LATC_LCNormalMaxLatAcc_ms2  ExtrapMethod=Clip  InternalRulePriority=Speed  RndMeth=Simplest  InputSameDT=on
  LC_CancelMaxAy : Lookup_n-D  NumberOfTableDimensions=1  BreakpointsForDimension1=P_LCS_VehicleSpd_TabX_Kph  Table=P_LCS_LATC_LCCancleMaxLatAcc_ms2  ExtrapMethod=Clip  InternalRulePriority=Speed  RndMeth=Simplest  InputSameDT=on
  LC_Eco_MaxAy : Lookup_n-D  NumberOfTableDimensions=1  BreakpointsForDimension1=P_LCS_VehicleSpd_TabX_Kph  Table=P_LCS_LATC_LCEcoMaxLatAcc_ms2  ExtrapMethod=Clip  InternalRulePriority=Speed  RndMeth=Simplest  InputSameDT=on
  LC_SportMaxAy : Lookup_n-D  NumberOfTableDimensions=1  BreakpointsForDimension1=P_LCS_VehicleSpd_TabX_Kph  Table=P_LCS_LATC_LCSportMaxLatAcc_ms2  ExtrapMethod=Clip  InternalRulePriority=Speed  RndMeth=Simplest  InputSameDT=on
  LKA Active : Lookup_n-D  NumberOfTableDimensions=1  BreakpointsForDimension1=P_LCS_VehicleSpd_TabX_Kph  Table=P_LCS_LATC_LKAAngleSlope_ratio  ExtrapMethod=Clip  InternalRulePriority=Speed  RndMeth=Simplest  InputSameDT=on
  LKA_MaxAy : Lookup_n-D  NumberOfTableDimensions=1  BreakpointsForDimension1=P_LCS_VehicleSpd_TabX_Kph  Table=P_LCS_LATC_LKAMaxLatAcc_ms2  ExtrapMethod=Clip  InternalRulePriority=Speed  RndMeth=Simplest  InputSameDT=on
  MATLAB Function3 : MATLAB Function  TreatAsAtomicUnit=on
  Merge : Merge
  Min : MinMax  Inputs=2
  Multiport Switch1 : MultiPortSwitch  DataPortOrder=Zero-based contiguous  Inputs=11  zeroidx=on
  Multiport Switch2 : MultiPortSwitch  DataPortOrder=Zero-based contiguous  Inputs=11  zeroidx=on
  No Function 2 LCK : Lookup_n-D  NumberOfTableDimensions=1  BreakpointsForDimension1=P_LCS_VehicleSpd_TabX_Kph  Table=P_LCS_LATC_LCKAngleSlope_ratio  ExtrapMethod=Clip  InternalRulePriority=Speed  RndMeth=Simplest  InputSameDT=on
  Product : Product
  Switch Case : SwitchCase  CaseConditions={[1,2,3,4,5]}
  Switch Case Action Subsystem : Subsystem  TreatAsAtomicUnit=on
  Switch Case Action Subsystem1 : Subsystem  TreatAsAtomicUnit=on
  Unit Delay3 : UnitDelay  SampleTime=-1  HasFrameUpgradeWarning=on
  Unit Delay4 : UnitDelay  SampleTime=-1  HasFrameUpgradeWarning=on
  Unit Delay5 : UnitDelay  SampleTime=-1  HasFrameUpgradeWarning=on
  VehSpd_kph1 : InportShadow  Port=2
  Max_Lateral_Acc : Outport  OutDataTypeStr=single
  SteerAngSlope : Outport  Port=2  OutDataTypeStr=single
  wires:
  Data Type Conversion1/1 -> SteerAngSlope/1
  Data Type Conversion/1 -> Max_Lateral_Acc/1
  LCNomal_MaxAy/1 -> Multiport Switch2/5
  LKA_MaxAy/1 -> Multiport Switch2/6
  LCKMaxAy/1 -> Multiport Switch2/3
  LCKIEMaxAy/1 -> Multiport Switch2/4
  ELK_MaxAy/1 -> Multiport Switch2/7
  VehSpd_kph1/1 -> LCKMaxAy/1, LCNomal_MaxAy/1, LC_CancelMaxAy/1, LC_SportMaxAy/1, LC_Eco_MaxAy/1, ESS AES_MaxAy/1, ELK_MaxAy/1, LKA_MaxAy/1, LCKIEMaxAy/1
  ESS AES_MaxAy/1 -> Multiport Switch2/8
  LC_Eco_MaxAy/1 -> Multiport Switch2/9
  LC_SportMaxAy/1 -> Multiport Switch2/10
  LC_CancelMaxAy/1 -> Multiport Switch2/11
  Constant5/1 -> Multiport Switch2/12
  Constant1/1 -> Multiport Switch2/2
  Multiport Switch2/1 -> Data Type Conversion/1  "LCS_LATC_MaxAy_ms2"
  LC Cancel/1 -> Multiport Switch1/11
  LCK/IE TO LC_Sport/1 -> Multiport Switch1/10
  LCK/IE TO LC_Eco/1 -> Multiport Switch1/9
  ESS AES Active/1 -> Multiport Switch1/8
  Unit Delay5/1 -> MATLAB Function3/3(TarDangerLevelK1)
  VehSpd_kph/1 -> LCKIE_Active/1, LKA Active/1, ELK Active/1, ESS AES Active/1, LCK/IE TO LC_Eco/1, LCK/IE TO LC_Sport/1, LC Cancel/1, LCK/IE TO LC_Nomal/1, No Function 2 LCK/1
  ELK Active/1 -> Multiport Switch1/7
  LCKIE_Active/1 -> Multiport Switch1/4
  Unit Delay3/1 -> MATLAB Function3/5(CntK1)
  Unit Delay4/1 -> MATLAB Function3/4(FLgK1)
  Constant/1 -> Multiport Switch1/2
  MATLAB Function3/2(Cnt) -> Product/2, Unit Delay3/1
  MATLAB Function3/1(FLg) -> Switch Case/1, Switch Case Action Subsystem/1(Flg), Unit Delay4/1  "LCS_LATC_AngleSlopeFlg_st"
  Constant2/1 -> MATLAB Function3/1(delytime)
  Multiport Switch1/1 -> Min/2  "LCS_LATC_StateAngleSlope_degs"
  No Function 2 LCK/1 -> Multiport Switch1/3
  LKA Active/1 -> Multiport Switch1/6
  Constant4/1 -> Multiport Switch1/12
  Constant3/1 -> Product/1
  Product/1 -> [HoldTime]  "LCS_LATC_HoldTime_s"
  Min/1 -> Data Type Conversion1/1
  LCK/IE TO LC_Nomal/1 -> Multiport Switch1/5
  Switch Case/1 -> Switch Case Action Subsystem/Action
  Switch Case/2 -> Switch Case Action Subsystem1/Action
  [HoldTime] -> Switch Case Action Subsystem/2(StateHoldTime)
  Switch Case Action Subsystem/1(Out1) -> Merge/2
  Switch Case Action Subsystem1/1(Out1) -> Merge/1
  Merge/1 -> Min/1  "LCS_LATC_StateActAngleSlope_degs"
  TarDangerlLevel/1 -> MATLAB Function3/2(TarDangerLevel), Unit Delay5/1, Multiport Switch2/1, Multiport Switch1/1

== system PvtSubSys_LATC/Subsystem/LateralControl/LCS_Angle/Lateral_Control/Dynamic_Model_LQR/Understeer&Offset_Calc ==
  note: %% 匀速
  SteerAngle_deg : Inport
  PsiDtOpt : Inport  Port=2
  axvRef : Inport  Port=3
  vxvRef : Inport  Port=4
  Abs2 : Abs
  Compare To Constant1 : simulink/Logic and Bit Operations/Compare To Constant  relop=>  const=P_LCS_LATC_CurOffsetVehicleSpdLimitValue_degs  OutDataTypeStr=boolean
  Compare To Constant6 : simulink/Logic and Bit Operations/Compare To Constant  relop=<=  const=1.5  OutDataTypeStr=boolean
  Constant1 : Constant  Value=P_Global_SteeringAngleRatio
  Constant4 : Constant  Value=P_Global_CharSpd_ms
  Constant5 : Constant  Value=P_Global_WheelBase_m
  Constant6 : Constant  Value=57.3  OutDataTypeStr=single
  Enabled Subsystem : Subsystem  TreatAsAtomicUnit=on
  FilterTime2 : Product  Inputs=*//  RndMeth=Zero
  Logical Operator : Logic  AllPortsSameDT=off  OutDataTypeStr=boolean
  Memory52 : Memory  InheritSampleTime=on
  Sum : Sum  Inputs=+-
  Terminator : Terminator
  YOD_Ackman : MATLAB Function  TreatAsAtomicUnit=on
  SteerAngleOffset_deg : Outport
  wires:
  SteerAngle_deg/1 -> FilterTime2/1
  Compare To Constant1/1 -> Logical Operator/2
  YOD_Ackman/2(PsiDtAck) -> Memory52/1, Sum/1
  Enabled Subsystem/1(SteerAngleOffset_deg) -> SteerAngleOffset_deg/1
  Constant5/1 -> YOD_Ackman/3(WheelBase)
  Constant4/1 -> YOD_Ackman/2(Vch)
  Memory52/1 -> YOD_Ackman/5(PsiDtAckK1)
  PsiDtOpt/1 -> Sum/2
  vxvRef/1 -> YOD_Ackman/1(VxvRef), Compare To Constant1/1
  Sum/1 -> Enabled Subsystem/2(Raw)
  Logical Operator/1 -> Enabled Subsystem/Enable, Terminator/1  "LCS_OffSetUpdate_Flg"
  Constant1/1 -> FilterTime2/2
  Constant6/1 -> FilterTime2/3
  YOD_Ackman/1(AckConst) -> Enabled Subsystem/1(AckConst)
  FilterTime2/1 -> YOD_Ackman/4(AlpWheelAngle)
  axvRef/1 -> Abs2/1
  Abs2/1 -> Compare To Constant6/1
  Compare To Constant6/1 -> Logical Operator/1
  [AbsRoadCurve] -> Enabled Subsystem/3(Curve)

== system PvtSubSys_LATC/Subsystem/LateralControl/LCS_Angle/Lateral_Control/MPC/Median_Filter ==
  In : Inport
  Constant11 : Constant  Value=P_LCS_LCC_TarAngleFliterWindowSize - single(2)  OutDataTypeStr=single
  Divide1 : Product  Inputs=*/
  Max of Elements1 : MinMax  Function=max
  MinMax2 : MinMax
  Minus1 : Sum  Inputs=--+
  Sum of Elements1 : Sum  Inputs=+
  Tapped Delay1 : simulink/Discrete/Tapped Delay  vinit=0.0  samptime=-1  NumDelays=P_LCS_LCC_TarAngleFliterWindowSize-1  DelayOrder=Newest  includeCurrent=on
  Out : Outport
  wires:
  Constant11/1 -> Divide1/2
  Tapped Delay1/1 -> Sum of Elements1/1, MinMax2/1, Max of Elements1/1
  Sum of Elements1/1 -> Minus1/3
  MinMax2/1 -> Minus1/1
  In/1 -> Tapped Delay1/1
  Minus1/1 -> Divide1/1
  Divide1/1 -> Out/1
  Max of Elements1/1 -> Minus1/2

== system PvtSubSys_LATC/Subsystem/LateralControl/LCS_Angle/Lateral_Control/MPC/Subsystem5 ==
  raw : Inport
  Slope : Inport  Port=2
  Add : Sum
  Add1 : Sum  Inputs=+-
  Max : MinMax  Inputs=2
  Min : MinMax  Function=max  Inputs=2
  Unit Delay : UnitDelay  InitialCondition=single(0)  SampleTime=-1  HasFrameUpgradeWarning=on
  out : Outport
  wires:
  Slope/1 -> Add1/2, Add/2
  Unit Delay/1 -> Add1/1, Add/1
  Min/1 -> out/1, Unit Delay/1
  Max/1 -> Min/1
  Add/1 -> Max/1
  Add1/1 -> Min/2
  raw/1 -> Max/2

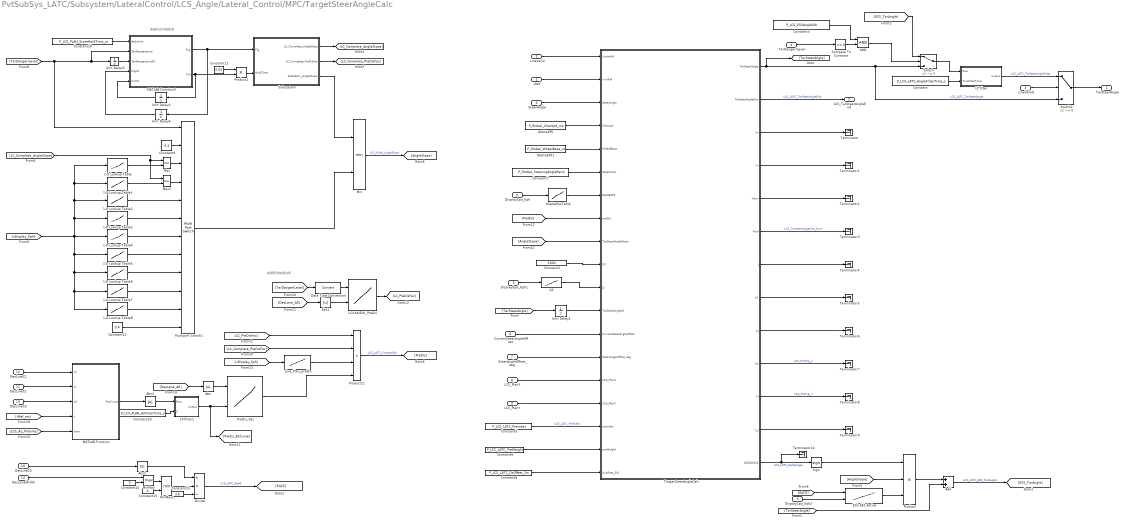
== system PvtSubSys_LATC/Subsystem/LateralControl/LCS_Angle/Lateral_Control/MPC/TargetSteerAngleCalc ==
  note: 换道状态切换检测
  note: 换道取消快速拉回
  vRef : Inport
  LineValid : Inport  Port=2
  TarDangerlLevel : Inport  Port=3
  SteerAngle : Inport  Port=4
  DisplaySpd_Kph : Inport  Port=5
  CurrentSteerAngleOffset : Inport  Port=6
  SteerAngleOffset_deg : Inport  Port=7
  LCS_PlanX : Inport  Port=8
  LCS_PlanY : Inport  Port=9
  DesLineC0 : Inport  Port=10
  DesLineC1 : Inport  Port=11
  DesLineC2 : Inport  Port=12
  DesLineC3 : Inport  Port=13
  DesLaneWidth : Inport  Port=14
  1-D Lookup Table : Lookup_n-D  NumberOfTableDimensions=1  BreakpointsForDimension1=P_LCS_LATC_VehicleSpd_TabX_Kph  Table=P_LCS_LATC_LCKAngleSlope_Tab_degs  InternalRulePriority=Speed  RndMeth=Simplest  InputSameDT=on
  1-D Lookup Table1 : Lookup_n-D  NumberOfTableDimensions=1  BreakpointsForDimension1=P_LCS_LATC_VehicleSpd_TabX_Kph  Table=P_LCS_LATC_LCKIEAngleSlope_Tab_degs  InternalRulePriority=Speed  RndMeth=Simplest  InputSameDT=on
  1-D Lookup Table2 : Lookup_n-D  NumberOfTableDimensions=1  BreakpointsForDimension1=P_LCS_LATC_VehicleSpd_TabX_Kph  Table=P_LCS_LATC_LCNormalAngleSlope_Tab_degs  InternalRulePriority=Speed  RndMeth=Simplest  InputSameDT=on
  1-D Lookup Table3 : Lookup_n-D  NumberOfTableDimensions=1  BreakpointsForDimension1=P_LCS_LATC_VehicleSpd_TabX_Kph  Table=P_LCS_LATC_LKAAngleSlope_Tab_degs  InternalRulePriority=Speed  RndMeth=Simplest  InputSameDT=on
  1-D Lookup Table4 : Lookup_n-D  NumberOfTableDimensions=1  BreakpointsForDimension1=P_LCS_LATC_VehicleSpd_TabX_Kph  Table=P_LCS_PLAN_ELKAngleSlope_Tab_degs  InternalRulePriority=Speed  RndMeth=Simplest  InputSameDT=on
  1-D Lookup Table5 : Lookup_n-D  NumberOfTableDimensions=1  BreakpointsForDimension1=P_LCS_LATC_VehicleSpd_TabX_Kph  Table=P_LCS_LATC_ESSAESAngleSlope_Tab_degs  InternalRulePriority=Speed  RndMeth=Simplest  InputSameDT=on
  1-D Lookup Table6 : Lookup_n-D  NumberOfTableDimensions=1  BreakpointsForDimension1=P_LCS_LATC_VehicleSpd_TabX_Kph  Table=P_LCS_LATC_LCEcoAngleSlope_Tab_degs  InternalRulePriority=Speed  RndMeth=Simplest  InputSameDT=on
  1-D Lookup Table7 : Lookup_n-D  NumberOfTableDimensions=1  BreakpointsForDimension1=P_LCS_LATC_VehicleSpd_TabX_Kph  Table=P_LCS_LATC_LCSportAngleSlope_Tab_degs  InternalRulePriority=Speed  RndMeth=Simplest  InputSameDT=on
  1-D Lookup Table8 : Lookup_n-D  NumberOfTableDimensions=1  BreakpointsForDimension1=P_LCS_LATC_VehicleSpd_TabX_Kph  Table=P_LCS_LATC_LCAngleSlope_Tab_degs  InternalRulePriority=Speed  RndMeth=Simplest  InputSameDT=on
  AND : Logic  AllPortsSameDT=off  OutDataTypeStr=boolean
  Abs{,1..2,4} (4 alike) : Abs
  Add : Sum
  Compare To Constant : simulink/Logic and Bit Operations/Compare To Constant  relop===  const=6  OutDataTypeStr=boolean
  Constant : Constant  Value=P_LCS_LATC_AngleFilterTime_s  OutDataTypeStr=single
  Constant1 : Constant  Value=1000  OutDataTypeStr=single
  Constant10 : Constant  Value=P_LCS_PLAN_StateHoldTime_st  OutDataTypeStr=uint16
  Constant11 : Constant  Value=0.02
  Constant12 : Constant  Value=0.4  OutDataTypeStr=single
  Constant13 : Constant  Value=3.6  OutDataTypeStr=single
  Constant14 : Constant  Value=3  OutDataTypeStr=single
  Constant15 : Constant  Value=4  OutDataTypeStr=single
  Constant20 : Constant  Value=P_LCS_PLAN_A2FliterTime_s
  Constant3 : Constant  Value=P_LCS_ESSAngleSW  OutDataTypeStr=boolean
  Constant5 : Constant  Value=P_LCS_LATC_Preindex  OutDataTypeStr=single
  Constant6 : Constant  Value=P_LCS_LATC_PreWeight  OutDataTypeStr=single
  Constant7 : Constant  Value=P_Global_SteeringAngleRatio  OutDataTypeStr=single
  Constant8 : Constant  Value=P_LCS_LATC_DxOffset_Sw
  Constant9 : Constant  Value=0.4  OutDataTypeStr=single
  Data Type Conversion : DataTypeConversion
  DisplaySpd_Kph1 : InportShadow  Port=5
  DisplaySpd_Kph2 : InportShadow  Port=5
  Divide : Product  Inputs=**/
  ESS AES Active : Lookup_n-D  BreakpointsForDimension1=P_LCS_LATC_ESSA0Dis_TabX_m  BreakpointsForDimension2=P_LCS_LATC_VehicleSpd_TabX_Kph  Table=P_LCS_LATC_ESSAddAngleSlope_Tab_degs  ExtrapMethod=Clip  UseLastTableValue=on  InternalRulePriority=Speed  OutDataTypeStr=single  RndMeth=Simplest
      settings: InputPortMap=u0,u1
  LC/LKA/ELK_PreDis : Lookup_n-D  BreakpointsForDimension1=P_LCS_PLAN_TarDangerlLevel_Tabx_st  BreakpointsForDimension2=P_LCS_PLAN_DesLineA0_TabY_m  Table=P_LCS_PLAN_LCPreDisFac_ratio  ExtrapMethod=Clip  UseLastTableValue=on  InternalRulePriority=Speed  RndMeth=Simplest  InputSameDT=on
      settings: InputPortMap=u0,u1
  LP filter : Subsystem
  LP filter1 : Subsystem
  LineValid1 : InportShadow  Port=2
  Line_Plan_preDis : Lookup_n-D  NumberOfTableDimensions=1  BreakpointsForDimension1=P_LCS_PLAN_VehicleSpd_TabX_Kph  Table=P_LCS_PLAN_PreDis_Tab_m  ExtrapMethod=Clip  UseLastTableValue=on  InternalRulePriority=Speed  RndMeth=Simplest  InputSameDT=on
  MATLAB Function : MATLAB Function  TreatAsAtomicUnit=on
  MATLAB Function3 : MATLAB Function  TreatAsAtomicUnit=on
  Max : MinMax  Function=max  Inputs=2
  Max1 : MinMax  Function=max  Inputs=2
  Min : MinMax  Inputs=2
  MinMax : MinMax  Function=max  Inputs=2
  MinMax1 : MinMax  Inputs=2
  Multiport Switch1 : MultiPortSwitch  DataPortOrder=Zero-based contiguous  Inputs=11  zeroidx=on
  PreDis_Fac : Lookup_n-D  BreakpointsForDimension1=P_LCS_PLAN_DesLineA0_TabX_m  BreakpointsForDimension2=P_LCS_PLAN_PreDisCurve_TabY_m  Table=P_LCS_PlLAN_PreDisFac_Tab_ratio  ExtrapMethod=Clip  UseLastTableValue=on  InternalRulePriority=Speed  RndMeth=Simplest  InputSameDT=on
      settings: InputPortMap=u0,u1
  Product : Product  Inputs=3  OutDataTypeStr=single
  Product1 : Product
  Product11 : Product  Inputs=4
  Q1 : Lookup_n-D  NumberOfTableDimensions=1  BreakpointsForDimension1=[0,5,10,15,20,25,30,35,40,60,80,90,100,110,120,140]  Table=[0,0,0,0,0,0,0,0,0,0,0,0,0,0,0,0]  InternalRulePriority=Speed  RndMeth=Simplest  InputSameDT=on
  Sign : Signum
  Subsystem : Subsystem
  Switch : Switch  Criteria=u2 ~= 0
  Switch2 : Switch  Criteria=u2 ~= 0
  TargetSteerAngleCalc : MATLAB Function  TreatAsAtomicUnit=on
  Terminator{,1..10} (11 alike) : Terminator
  Unit Delay{1,3..5} (4 alike) : UnitDelay  SampleTime=-1  HasFrameUpgradeWarning=on
  tDeltaEPS : Constant  Value=P_Global_CharSpd_ms
  tDeltaEPS1 : Constant  Value=P_Global_WheelBase_m
  tDeltaEpsTable : Lookup_n-D  NumberOfTableDimensions=1  BreakpointsForDimension1=P_LCS_PLAN_VehicleSpd_TabX_Kph  Table=P_LCS_LATC_DeltaEps_Tab_s  ExtrapMethod=Clip  InternalRulePriority=Speed  RndMeth=Simplest  InputSameDT=on
  TarSteerAngle : Outport
  LCS_TarSteerAngleEnd : Outport  Port=2
  wires:
  Constant8/1 -> TargetSteerAngleCalc/19(dxoffset_SW)
  Constant6/1 -> TargetSteerAngleCalc/18(preWeight)
  Constant5/1 -> TargetSteerAngleCalc/17(preindex)  "LCS_LATC_PreIndex"
  LCS_PlanY/1 -> TargetSteerAngleCalc/16(LCS_PlanY)
  LCS_PlanX/1 -> TargetSteerAngleCalc/15(LCS_PlanX)
  LineValid1/1 -> Switch2/2
  ESS AES Active/1 -> Product/3
  DisplaySpd_Kph2/1 -> ESS AES Active/2
  [EqC0] -> ESS AES Active/1
  TarDangerlLevel/1 -> Compare To Constant/1
  TargetSteerAngleCalc/13(ADDANGLE) -> Sign/1, Terminator10/1  "LCS_LATC_DeltaAngle"
  Sign/1 -> Product/1
  [AngleSlope] -> Product/2
  Product/1 -> Add/1
  [TarSteerAngle] -> Add/2
  Add/1 -> [ESS_TarAngle]  "LCS_LATC_ESS_TarAngle2"
  TargetSteerAngleCalc/1(TarSteerAngle) -> Switch/3, Switch2/3, [TarSteerAngle]  "LCS_LATC_TarSteerAngle"
  Constant/1 -> LP filter/2(TorqFilterTime)
  LP filter/1(output) -> Switch2/1  "LCS_LATC_TarSteerAngleFilter"
  Switch/1 -> LP filter/1(Raw)
  [ESS_TarAngle] -> Switch/1
  Constant3/1 -> AND/1
  Compare To Constant/1 -> AND/2
  AND/1 -> Switch/2
  Switch2/1 -> TarSteerAngle/1
  TargetSteerAngleCalc/12(t_y) -> Terminator9/1
  TargetSteerAngleCalc/2(TarSteerAngleEnd) -> LCS_TarSteerAngleEnd/1  "LCS_LATC_TarSteerAngleEnd"
  [PreDis] -> TargetSteerAngleCalc/8(preDis)
  [AngleSlope] -> TargetSteerAngleCalc/9(TarSteerAngleSlope)
  SteerAngle/1 -> TargetSteerAngleCalc/3(SteerAngle)
  vRef/1 -> TargetSteerAngleCalc/2(vxvRef)
  TargetSteerAngleCalc/11(YY) -> Terminator8/1  "LCS_PreTraj_Y"
  TargetSteerAngleCalc/10(XX) -> Terminator7/1  "LCS_PreTraj_X"
  Constant1/1 -> TargetSteerAngleCalc/10(R1)
  TargetSteerAngleCalc/9(Jq) -> Terminator6/1
  TargetSteerAngleCalc/8(Jr1) -> Terminator5/1
  TargetSteerAngleCalc/7(J) -> Terminator4/1
  TargetSteerAngleCalc/6(Num) -> Terminator3/1  "LCS_TarSteerAngleCalc_Num"
  TargetSteerAngleCalc/5(Yawn) -> Terminator2/1
  TargetSteerAngleCalc/4(Yn) -> Terminator1/1
  TargetSteerAngleCalc/3(Xn) -> Terminator/1
  Constant7/1 -> TargetSteerAngleCalc/6(SteerRatio)
  tDeltaEpsTable/1 -> TargetSteerAngleCalc/7(tDeltaEPS)
  DisplaySpd_Kph/1 -> tDeltaEpsTable/1
  tDeltaEPS/1 -> TargetSteerAngleCalc/4(Charspd)
  tDeltaEPS1/1 -> TargetSteerAngleCalc/5(WheelBase)
  [TarSteerAngle] -> Unit Delay1/1
  Unit Delay1/1 -> TargetSteerAngleCalc/12(TarSteerAngleK1)
  Q1/1 -> TargetSteerAngleCalc/11(Q)
  DisplaySpd_Kph1/1 -> Q1/1
  CurrentSteerAngleOffset/1 -> TargetSteerAngleCalc/13(CurrentSteerAngleOffset)
  LineValid/1 -> TargetSteerAngleCalc/1(LineValid)
  SteerAngleOffset_deg/1 -> TargetSteerAngleCalc/14(SteerAngleOffset_deg)
  Constant12/1 -> Multiport Switch1/12
  1-D Lookup Table7/1 -> Multiport Switch1/10
  MATLAB Function3/1(FLg) -> Unit Delay4/1, Subsystem/1(Flg)
  MATLAB Function3/2(Cnt) -> Product1/2, Unit Delay3/1
  Unit Delay3/1 -> MATLAB Function3/5(CntK1)
  1-D Lookup Table4/1 -> Multiport Switch1/7
  1-D Lookup Table/1 -> Max/2
  Unit Delay5/1 -> MATLAB Function3/3(TarDangerLevelK1)
  1-D Lookup Table2/1 -> Multiport Switch1/5
  1-D Lookup Table5/1 -> Multiport Switch1/8
  1-D Lookup Table6/1 -> Multiport Switch1/9
  Max1/1 -> Multiport Switch1/4
  Max/1 -> Multiport Switch1/3
  [LC_Complete_AngleSlope] -> Max1/1, Max/1
  [TarDangerlLevel] -> MATLAB Function3/2(TarDangerLevel), Unit Delay5/1, Multiport Switch1/1
  Constant9/1 -> Multiport Switch1/2
  Constant10/1 -> MATLAB Function3/1(delytime)
  1-D Lookup Table3/1 -> Multiport Switch1/6
  Product1/1 -> Subsystem/2(HoldTime)
  1-D Lookup Table8/1 -> Multiport Switch1/11
  Min/1 -> [AngleSlope]  "LCS_PLAN_AngleSlope"
  Unit Delay4/1 -> MATLAB Function3/4(FLgK1)
  Multiport Switch1/1 -> Min/2
  1-D Lookup Table1/1 -> Max1/2
  Constant11/1 -> Product1/1
  PreDis_Fac/1 -> Product11/4
  Line_Plan_preDis/1 -> Product11/3
  MATLAB Function/1(PreCurve) -> Abs4/1
  DesLineC2/1 -> MATLAB Function/1(c2)
  [vRef_ms] -> MATLAB Function/4(v)
  Data Type Conversion/1 -> LC/LKA/ELK_PreDis/1
  Abs/1 -> PreDis_Fac/1
  [DesLane_A0] -> Abs1/1
  Abs1/1 -> LC/LKA/ELK_PreDis/2
  [vDisplay_Kph] -> Line_Plan_preDis/1
  LC/LKA/ELK_PreDis/1 -> [LC_PreDisFac]
  [TarDangerlLevel] -> Data Type Conversion/1
  [DesLane_A0] -> Abs/1
  DesLineC3/1 -> MATLAB Function/3(c3)
  Constant20/1 -> LP filter1/2(TorqFilterTime)
  Abs4/1 -> LP filter1/1(Raw)
  Product11/1 -> [PreDis]  "LCS_LATC_FinalpreDis"
  [LC_PreDisFac] -> Product11/1
  LP filter1/1(output) -> PreDis_Fac/2, [Predis_A2Curve]
  [LC_Complete_PreDisFac] -> Product11/2
  [LCS_A2_Pretime] -> MATLAB Function/5(time)
  DesLineC1/1 -> MATLAB Function/2(c1)
  [vDisplay_Kph] -> 1-D Lookup Table8/1, 1-D Lookup Table7/1, 1-D Lookup Table6/1, 1-D Lookup Table5/1, 1-D Lookup Table2/1, 1-D Lookup Table1/1, 1-D Lookup Table/1, 1-D Lookup Table3/1, 1-D Lookup Table4/1
  Subsystem/1(LC_Complete_AngleSlope) -> [LC_Complete_AngleSlope]
  Subsystem/3(StateActiv_AngleSlope) -> Min/1
  Subsystem/2(LC_Complete_PreDisFac) -> [LC_Complete_PreDisFac]
  Constant15/1 -> MinMax1/2
  Constant13/1 -> Divide/3
  MinMax1/1 -> Divide/2
  DesLineC0/1 -> Abs2/1
  MinMax/1 -> MinMax1/1
  Divide/1 -> [EqC0]  "LCS_LATC_EqA0"
  Constant14/1 -> MinMax/2
  DesLaneWidth/1 -> MinMax/1
  Abs2/1 -> Divide/1
